simulink model "blance_leg2"  (R2021b)
settings: Solver=VariableStepAuto  StartTime=0.0  StopTime=10  RelTol=1e-3
values from neighbouring files (symbols this model uses):
  K = get_k_length(0.14)    [get_k.m]    (also in get_k_length.m = lqr(A,B,Q,R))
  N = NM + mp*diff(x + L*sin(theta),t,2)    [get_k_length.m]
undefined symbols (not defined in the file or in its folder): X, Y, Z
libraries: sm_lib x76, nesl_utility x25, slpidlib x2
(part 1 of 3)
settings Model: Creator=Hhop  LastModifiedBy=34511
settings SolverCC: AlgebraicLoopSolver=TrustRegion  MinimalZcImpactIntegration=on
settings DebuggingCC: ReadBeforeWriteMsg=DisableAll  WriteAfterWriteMsg=DisableAll  WriteAfterReadMsg=DisableAll  MultiTaskDSMMsg=none  UnconnectedInputMsg=none  UnconnectedOutputMsg=none  UnconnectedLineMsg=none
settings ModelReferenceCC: UpdateModelReferenceTargets=IfOutOfDate  EnableRefExpFcnMdlSchedulingChecks=off
settings SFSimCC: SFSimEcho=off

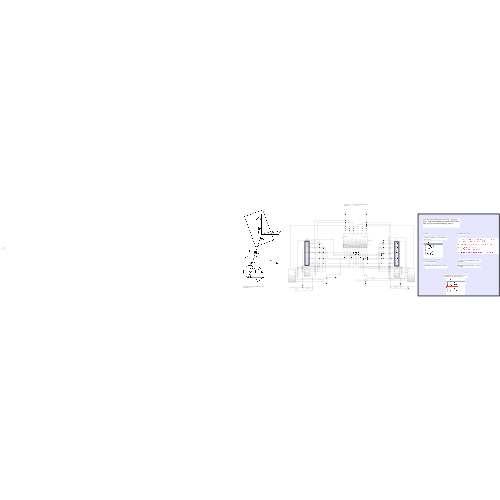
[thumbnail: Simulink's stored preview of the top-level diagram]
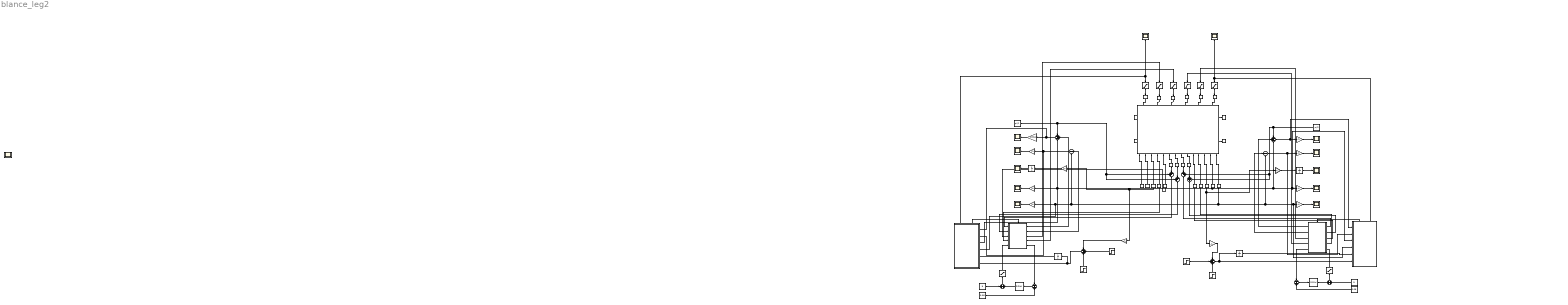
== system blance_leg2 ==
  note: 参考开源文档作者：韭菜的菜 链接：https://zhuanlan.zhihu.com/p/613007726 来源：知乎
  note: 图片来源 韭菜的菜 链接：https://zhuanlan.zhihu.com/p/613007726来源：知乎
  note: 运行步骤 :
  note: 所有开源文件必须置于同一文件夹(最好不要使用中文路径)
  note: 得到K参数后进入simulink 点击“运行”开始仿真
  note: addpath'(你所要想添加到的路径)'，具体用法可自行搜索
  note: 如果遇到如下图所示错误
  note: 可点击将其文件夹添加到MATLAB，或输入代码更换路径
  note: K = get_k_length(0.08)
  note: 在命令行窗口运行下图所示代码
  note: 如果想获取K矩阵关于腿长的函数的三次多项式系数在命令行窗口运行下图所示文件
  note: 该仿真是在b站轮腿机器人仿真开源上进行修改，链接：https://www.bilibili.com/read/cv26677904/?spm_id_from=333.999.0.0&jump_opus=1
  Constant : Constant  Value=0.08
  Constant1 : Constant  Value=0.08
  Constant10 : Constant  Value=pi/2
  Constant12 : Constant  Value=pi/2
  Gain{,1,29,41} (4 alike) : Gain  Gain=-0.0603
  Gain{22,24..26,33,36,38,40} (8 alike) : Gain  Gain=180/pi
  Integrator{1..4} (4 alike) : Integrator
  L_X : Scope
  L_d_phi : Scope
  L_d_theta : Scope
  L_phi : Scope
  L_theta : Scope
  PID Controller2 : slpidlib/PID Controller  Controller=PID  Form=Parallel  TimeDomain=Continuous-time  UseExternalTs=off  SampleTime=-1  IntegratorMethod=Forward Euler  FilterMethod=Forward Euler  ControllerParametersSource=internal  P=220  I=0  D=1000  UseFilter=on  N=100  TunerSelectOption=Transfer Function Based (PID Tuner App)  InitialConditionSource=internal  InitialConditionForIntegrator=0  InitialConditionForFilter=0  DifferentiatorICPrevScaledInput=0  ExternalReset=none  TrackingMode=off  Kt=1  LimitOutput=off  SatLimitsSource=internal  UpperSaturationLimit=inf  LowerSaturationLimit=-inf  LinearizeAsGain=on  AntiWindupMode=none  Kb=1  POutMin=[]  POutMax=[]  IOutMin=[]  IOutMax=[]  DOutMin=[]  DOutMax=[]  NOutMin=[]  NOutMax=[]  SumOutMin=[]  SumOutMax=[]  SaturationOutMin=[]  SaturationOutMax=[]  PParamMin=[]  PParamMax=[]  IParamMin=[]  IParamMax=[]  DParamMin=[]  DParamMax=[]  NParamMin=[]  NParamMax=[]  KbParamMin=[]  KbParamMax=[]  KtParamMin=[]  KtParamMax=[]  KbOutMin=[]  KbOutMax=[]  KtOutMin=[]  KtOutMax=[]  IntegratorOutMin=[]  IntegratorOutMax=[]  FilterOutMin=[]  FilterOutMax=[]  SumI1OutMin=[]  SumI1OutMax=[]  SumI2OutMin=[]  SumI2OutMax=[]  SumI3OutMin=[]  SumI3OutMax=[]  SumI4OutMin=[]  SumI4OutMax=[]  SumDOutMin=[]  SumDOutMax=[]  DifferentiatorOutMin=[]  DifferentiatorOutMax=[]  FilterDiffOutCoefMin=[]  FilterDiffOutCoefMax=[]  ReciprocalOutMin=[]  ReciprocalOutMax=[]  SumDenOutMin=[]  SumDenOutMax=[]  SumNumOutMin=[]  SumNumOutMax=[]  DivideOutMin=[]  DivideOutMax=[]  UdiffTsProdOutMin=[]  UdiffTsProdOutMax=[]  NTsProdOutMin=[]  NTsProdOutMax=[]  UintegralTsProdOutMin=[]  UintegralTsProdOutMax=[]  UngainTsProdOutMin=[]  UngainTsProdOutMax=[]  IntegratorContinuousStateAttributes=''  IntegratorStateMustResolveToSignalObject=off  IntegratorRTWStateStorageClass=Auto  FilterContinuousStateAttributes=''  FilterStateMustResolveToSignalObject=off  FilterRTWStateStorageClass=Auto  ParallelPVariant=InternalParameters  IdealPVariant=Disabled  IVariant=InternalParameters  DVariant=InternalParameters  IntegratorVariant=Continuous  SatVariant=Disabled  AWVariant=Passthrough  PCopyVariant=Disabled  TRVariant=Disabled  FdbkBlocksVariant=Forward  IdealPFdbkVariant=Disabled  SatFdbkVariant=Disabled  DerivativeFilterVariant=ContFilter  NVariant=InternalParameters  NCopyVariant=Disabled  FilterICVariant=InternalICsFilter  IntegratorICVariant=InternalICs  ExternalResetVariant=Disabled  TRSumVariant=Passthrough  SumFdbkVariant=Disabled  SumVariant=Sum_PID  TsampFilterVariant=InternalTs  TsampNgainVariant=Passthrough  TsampIntegralVariant=Passthrough  ExternalSaturationOutDataTypeStr=Inherit: Same as second input
  PID Controller3 : slpidlib/PID Controller  Controller=PID  Form=Parallel  TimeDomain=Continuous-time  UseExternalTs=off  SampleTime=-1  IntegratorMethod=Forward Euler  FilterMethod=Forward Euler  ControllerParametersSource=internal  P=220  I=0  D=1000  UseFilter=on  N=100  TunerSelectOption=Transfer Function Based (PID Tuner App)  InitialConditionSource=internal  InitialConditionForIntegrator=0  InitialConditionForFilter=0  DifferentiatorICPrevScaledInput=0  ExternalReset=none  TrackingMode=off  Kt=1  LimitOutput=off  SatLimitsSource=internal  UpperSaturationLimit=inf  LowerSaturationLimit=-inf  LinearizeAsGain=on  AntiWindupMode=none  Kb=1  POutMin=[]  POutMax=[]  IOutMin=[]  IOutMax=[]  DOutMin=[]  DOutMax=[]  NOutMin=[]  NOutMax=[]  SumOutMin=[]  SumOutMax=[]  SaturationOutMin=[]  SaturationOutMax=[]  PParamMin=[]  PParamMax=[]  IParamMin=[]  IParamMax=[]  DParamMin=[]  DParamMax=[]  NParamMin=[]  NParamMax=[]  KbParamMin=[]  KbParamMax=[]  KtParamMin=[]  KtParamMax=[]  KbOutMin=[]  KbOutMax=[]  KtOutMin=[]  KtOutMax=[]  IntegratorOutMin=[]  IntegratorOutMax=[]  FilterOutMin=[]  FilterOutMax=[]  SumI1OutMin=[]  SumI1OutMax=[]  SumI2OutMin=[]  SumI2OutMax=[]  SumI3OutMin=[]  SumI3OutMax=[]  SumI4OutMin=[]  SumI4OutMax=[]  SumDOutMin=[]  SumDOutMax=[]  DifferentiatorOutMin=[]  DifferentiatorOutMax=[]  FilterDiffOutCoefMin=[]  FilterDiffOutCoefMax=[]  ReciprocalOutMin=[]  ReciprocalOutMax=[]  SumDenOutMin=[]  SumDenOutMax=[]  SumNumOutMin=[]  SumNumOutMax=[]  DivideOutMin=[]  DivideOutMax=[]  UdiffTsProdOutMin=[]  UdiffTsProdOutMax=[]  NTsProdOutMin=[]  NTsProdOutMax=[]  UintegralTsProdOutMin=[]  UintegralTsProdOutMax=[]  UngainTsProdOutMin=[]  UngainTsProdOutMax=[]  IntegratorContinuousStateAttributes=''  IntegratorStateMustResolveToSignalObject=off  IntegratorRTWStateStorageClass=Auto  FilterContinuousStateAttributes=''  FilterStateMustResolveToSignalObject=off  FilterRTWStateStorageClass=Auto  ParallelPVariant=InternalParameters  IdealPVariant=Disabled  IVariant=InternalParameters  DVariant=InternalParameters  IntegratorVariant=Continuous  SatVariant=Disabled  AWVariant=Passthrough  PCopyVariant=Disabled  TRVariant=Disabled  FdbkBlocksVariant=Forward  IdealPFdbkVariant=Disabled  SatFdbkVariant=Disabled  DerivativeFilterVariant=ContFilter  NVariant=InternalParameters  NCopyVariant=Disabled  FilterICVariant=InternalICsFilter  IntegratorICVariant=InternalICs  ExternalResetVariant=Disabled  TRSumVariant=Passthrough  SumFdbkVariant=Disabled  SumVariant=Sum_PID  TsampFilterVariant=InternalTs  TsampNgainVariant=Passthrough  TsampIntegralVariant=Passthrough  ExternalSaturationOutDataTypeStr=Inherit: Same as second input
  PS-Simulink Converter{1,18..22,24,27..37} (18 alike) : nesl_utility/PS-Simulink Converter  PhysicalDomain=network_engine_domain  SubClassName=ps_output  LeftPortType=input  RightPortType=output  PseudoPeriodic=off  Frequencies=[]  Unit=inherit  AffineConversion=off
      settings: SourceProductBaseCode=PW,SS
  R_X : Scope
  R_d_phi : Scope
  R_d_theta : Scope
  R_phi : Scope
  R_theta : Scope
  Saturation{1..4} (4 alike) : Saturate  UpperLimit=100  LowerLimit=-100
  Saturation5 : Saturate  UpperLimit=300  LowerLimit=-300
  Saturation6 : Saturate  UpperLimit=300  LowerLimit=-300
  Saturation7 : Saturate  UpperLimit=9  LowerLimit=-9
  Saturation8 : Saturate  UpperLimit=9  LowerLimit=-9
  Scope1 : Scope
  Scope6 : Scope
  Simulink-PS Converter{1..6} (6 alike) : nesl_utility/Simulink-PS Converter  PhysicalDomain=network_engine_domain  SubClassName=ps_input  LeftPortType=input  RightPortType=output  PseudoPeriodic=off  Frequencies=[]  NoiseDistribution=none  NoiseParameters=[]  Unit=1  AffineConversion=off  FilteringAndDerivatives=provide  SimscapeFilterOrder=1  InputFilterTimeConstant=0.001  UdotUserProvided=0
      settings: SourceProductBaseCode=PW,SS
  Step1 : Step  Time=2  After=0.5  SampleTime=0
  Step5 : Step  Time=5  After=0.5  SampleTime=0
  Step6 : Step  Time=5  After=0.5  SampleTime=0
  Step7 : Step  Time=2  After=0.5  SampleTime=0
  Subsystem1 : Subsystem
      settings: PortSchema="{\"entries\":[{\"content\":{\"sides\":[{\"content\":{\"connectorIds\":[\"In1\",\"In2\",\"In3\",\"In4\",\"In5\",\"In6\"]},\"type\":\"ConnectorPlacement.EquallySpacedRectSide\",\"uuid\":\"055cb80c-cd03-4a8d-aef8-6b3df8c72d3f\"},{\"content\":{\"connectorIds\":[],\"side\":\"RIGHT\"},\"type\":\"ConnectorPlacement.EquallySpacedRectSide\",\"uuid\":\"5756fad1-d70f-4a11-a5af-d2f67bfb0d7e\"},{\"content\":{\"connectorIds\":[\"Out1\",\"Out2\"],\"side\":\"TOP\"},\"type\":\"ConnectorPlacement.EquallySpacedRectSide\",\"uuid\":\"9c70cf42-10f8-4525-9406-562484abf580\"}]},\"type\":\"ConnectorPlacement.EquallySpacedConnector\",\"uuid\":\"7084d402-0e44-4d2f-8cc2-1336d196e84d\"}],\"packageUris\":[\"http://schema.mathworks.com/mf0/Connector/R2020b\"],\"version\":\"1.0\"}"
  Subsystem4 : Subsystem
      settings: PortSchema="{\"entries\":[{\"content\":{\"sides\":[{\"content\":{\"connectorIds\":[\"In1\",\"In2\",\"In3\",\"In4\",\"In5\"]},\"type\":\"ConnectorPlacement.EquallySpacedRectSide\",\"uuid\":\"40de31e0-cc19-460f-99e9-affbb47f7204\"},{\"content\":{\"connectorIds\":[\"Out1\",\"Out2\",\"Out3\",\"Out4\",\"Out5\"],\"side\":\"RIGHT\"},\"type\":\"ConnectorPlacement.EquallySpacedRectSide\",\"uuid\":\"e61df4ab-633d-456a-aa2d-223df880274d\"},{\"content\":{\"connectorIds\":[\"In6\"],\"side\":\"TOP\"},\"type\":\"ConnectorPlacement.EquallySpacedRectSide\",\"uuid\":\"a7334146-3144-4ab1-9f08-8bf1583597b4\"}]},\"type\":\"ConnectorPlacement.EquallySpacedConnector\",\"uuid\":\"1490fe93-b025-4c86-96e6-b1bfc13c7f50\"}],\"packageUris\":[\"http://schema.mathworks.com/mf0/Connector/R2020b\"],\"version\":\"1.0\"}"
  Sum1 : Sum  Inputs=+-+
  Sum13 : Sum  Inputs=++|
  Sum14 : Sum  Inputs=|++
  Sum15 : Sum  Inputs=|++
  Sum16 : Sum  Inputs=|--
  Sum17 : Sum  Inputs=+--
  Sum18 : Sum  Inputs=+|+
  Sum2 : Sum  Inputs=+-+
  Sum20 : Sum  Inputs=++|
  Sum23 : Sum  Inputs=-|+
  Sum24 : Sum  Inputs=+--
  Sum25 : Sum  Inputs=+|+
  Sum27 : Sum  Inputs=|--
  Sum29 : Sum  Inputs=-|+
  blance_leg_model : Subsystem
      settings: PortSchema="{\"entries\":[{\"content\":{\"sides\":[{\"content\":{\"connectorIds\":[\"LConn1\",\"LConn2\",\"LConn3\",\"LConn4\",\"LConn5\",\"LConn6\"]},\"type\":\"ConnectorPlacement.EquallySpacedRectSide\",\"uuid\":\"df2d0b15-ec70-4430-8d90-67c6d88950b4\"},{\"content\":{\"connectorIds\":[\"RConn1\",\"RConn2\",\"RConn3\",\"RConn4\",\"RConn5\",\"RConn6\",\"RConn7\",\"RConn8\",\"RConn9\",\"RConn10\",\"RConn11\",\"RConn12\",\"RConn13\",\"RConn14\"],\"side\":\"RIGHT\"},\"type\":\"ConnectorPlacement.EquallySpacedRectSide\",\"uuid\":\"ec9b4787-d265-4ad9-b676-e253d2304993\"},{\"content\":{\"connectorIds\":[\"LConn7\",\"LConn8\"],\"side\":\"TOP\"},\"type\":\"ConnectorPlacement.EquallySpacedRectSide\",\"uuid\":\"40dd08fe-dc32-4cee-bbb8-c1ec6d04ee32\"},{\"content\":{\"connectorIds\":[\"RConn15\",\"RConn16\"],\"side\":\"BOTTOM\"},\"type\":\"ConnectorPlacement.EquallySpacedRectSide\",\"uuid\":\"0f9c1faf-3e52-4dca-bbb1-0993be9fa88c\"}]},\"type\":\"ConnectorPlacement.EquallySpacedConnector\",\"uuid\":\"d540d646-85aa-4f97-ae4d-1bccec971368\"}],\"packageUris\":[\"http://schema.mathworks.com/mf0/Connector/R2020b\"],\"version\":\"1.0\"}"
  calc : Subsystem
      settings: PortSchema="{\"entries\":[{\"content\":{\"sides\":[{\"content\":{\"connectorIds\":[\"In1\",\"In2\",\"In3\",\"In4\",\"In5\",\"In6\"]},\"type\":\"ConnectorPlacement.EquallySpacedRectSide\",\"uuid\":\"055cb80c-cd03-4a8d-aef8-6b3df8c72d3f\"},{\"content\":{\"connectorIds\":[],\"side\":\"RIGHT\"},\"type\":\"ConnectorPlacement.EquallySpacedRectSide\",\"uuid\":\"5756fad1-d70f-4a11-a5af-d2f67bfb0d7e\"},{\"content\":{\"connectorIds\":[\"Out1\",\"Out2\"],\"side\":\"TOP\"},\"type\":\"ConnectorPlacement.EquallySpacedRectSide\",\"uuid\":\"9c70cf42-10f8-4525-9406-562484abf580\"}]},\"type\":\"ConnectorPlacement.EquallySpacedConnector\",\"uuid\":\"7084d402-0e44-4d2f-8cc2-1336d196e84d\"}],\"packageUris\":[\"http://schema.mathworks.com/mf0/Connector/R2020b\"],\"version\":\"1.0\"}"
  control : Subsystem
      settings: PortSchema="{\"entries\":[{\"content\":{\"sides\":[{\"content\":{\"connectorIds\":[\"In1\",\"In2\",\"In3\",\"In4\",\"In5\"]},\"type\":\"ConnectorPlacement.EquallySpacedRectSide\",\"uuid\":\"40de31e0-cc19-460f-99e9-affbb47f7204\"},{\"content\":{\"connectorIds\":[\"Out1\",\"Out2\",\"Out3\",\"Out4\",\"Out5\"],\"side\":\"RIGHT\"},\"type\":\"ConnectorPlacement.EquallySpacedRectSide\",\"uuid\":\"e61df4ab-633d-456a-aa2d-223df880274d\"},{\"content\":{\"connectorIds\":[\"In6\"],\"side\":\"TOP\"},\"type\":\"ConnectorPlacement.EquallySpacedRectSide\",\"uuid\":\"a7334146-3144-4ab1-9f08-8bf1583597b4\"}]},\"type\":\"ConnectorPlacement.EquallySpacedConnector\",\"uuid\":\"1490fe93-b025-4c86-96e6-b1bfc13c7f50\"}],\"packageUris\":[\"http://schema.mathworks.com/mf0/Connector/R2020b\"],\"version\":\"1.0\"}"
  mean_x2 : Scope
  除去轮子后机体重量 : Constant  Value=9
  除去轮子后机体重量， : Constant  Value=9
  wires:
  Integrator4/1 -> R_X/1  "x"
  Integrator2/1 -> L_X/1  "x"
  除去轮子后机体重量，/1 -> Sum25/1
  Sum27/1 -> Subsystem1/2(d_theta), Gain25/1
  Gain40/1 -> L_d_phi/1
  Gain24/1 -> R_theta/1
  Gain38/1 -> L_d_theta/1
  Constant12/1 -> Sum15/2, Sum14/2, Sum17/1
  Sum29/1 -> PID Controller3/1
  Gain33/1 -> R_phi/1
  Gain36/1 -> L_theta/1
  Gain41/1 -> Integrator2/1  "x'"
  Sum16/1 -> calc/2(d_theta), Gain38/1
  Gain26/1 -> R_d_phi/1
  Constant/1 -> Sum29/2
  Gain22/1 -> L_phi/1
  Sum24/1 -> calc/1(theta), Gain36/1
  Constant10/1 -> Sum20/1, Sum13/1, Sum24/1
  Gain29/1 -> Integrator4/1  "x'"
  Sum23/1 -> PID Controller2/1
  PID Controller2/1 -> Sum25/2
  Sum17/1 -> Subsystem1/1(theta), Gain24/1
  Gain25/1 -> R_d_theta/1
  除去轮子后机体重量/1 -> Sum18/2
  PID Controller3/1 -> Sum18/1
  Saturation1/1 -> Simulink-PS Converter1/1
  Saturation2/1 -> Simulink-PS Converter3/1
  Saturation3/1 -> Simulink-PS Converter2/1
  Saturation4/1 -> Simulink-PS Converter5/1
  PS-Simulink Converter32/1 -> Sum13/2
  PS-Simulink Converter35/1 -> Sum15/1
  PS-Simulink Converter33/1 -> Sum14/1
  PS-Simulink Converter34/1 -> Sum20/2
  Sum13/1 -> control/1(phi1)
  Sum20/1 -> control/2(phi4)
  Sum14/1 -> Subsystem4/1(phi1)
  Sum15/1 -> Subsystem4/2(phi4)
  PS-Simulink Converter31/1 -> control/3(d_phi1)
  PS-Simulink Converter29/1 -> control/4(d_phi4)
  PS-Simulink Converter20/1 -> Subsystem4/3(d_phi1)
  PS-Simulink Converter21/1 -> Subsystem4/4(d_phi4)
  PS-Simulink Converter28/1 -> Gain41/1, Gain1/1
  PS-Simulink Converter22/1 -> Gain29/1, Gain/1
  PS-Simulink Converter1/1 -> calc/3(phi), Gain22/1, Sum24/3, Subsystem1/3(phi), Gain33/1, Sum17/3
  PS-Simulink Converter24/1 -> calc/4(d_phi), Gain40/1, Sum16/2, Subsystem1/4(d_phi), Gain26/1, Sum27/2
  control/5(L0) -> Sum23/1
  control/1(phi0) -> Sum24/2
  control/2(d_phi0) -> Sum16/1
  Subsystem4/1(phi0) -> Sum17/2
  Subsystem4/2(d_phi0) -> Sum27/1
  Subsystem4/5(L0) -> Sum29/1
  calc/1(Tp) -> control/6(Tp)
  Sum18/1 -> Saturation5/1
  Sum25/1 -> Saturation6/1
  Saturation6/1 -> control/5(F0)
  Constant1/1 -> Sum23/2
  control/3(T1) -> Saturation1/1
  Subsystem4/3(T1) -> Saturation4/1
  control/4(T2) -> Saturation2/1
  Subsystem4/4(T2) -> Saturation3/1
  calc/2(T) -> Saturation7/1, Scope1/1
  Subsystem1/2(T) -> Saturation8/1, Scope6/1
  Saturation7/1 -> Simulink-PS Converter6/1
  Saturation8/1 -> Simulink-PS Converter4/1
  Integrator1/1 -> Subsystem1/5(x)
  Integrator3/1 -> calc/5(x)
  Gain1/1 -> Sum1/1
  Sum1/1 -> calc/6(d_x), Integrator3/1
  Gain/1 -> Sum2/1
  Sum2/1 -> Integrator1/1, Subsystem1/6(d_x)
  Step1/1 -> Sum1/2
  Step5/1 -> Sum1/3
  Step7/1 -> Sum2/2
  Step6/1 -> Sum2/3
  Subsystem1/1(Tp) -> Subsystem4/6(Tp)
  Saturation5/1 -> Subsystem4/5(F0)
  connections:
  blance_leg_model/LConn2 -- Simulink-PS Converter1/RConn1
  blance_leg_model/LConn3 -- Simulink-PS Converter3/RConn1
  blance_leg_model/LConn4 -- Simulink-PS Converter2/RConn1
  blance_leg_model/LConn5 -- Simulink-PS Converter5/RConn1
  blance_leg_model/RConn10 -- PS-Simulink Converter20/LConn1
  blance_leg_model/RConn11 -- PS-Simulink Converter21/LConn1
  blance_leg_model/RConn2 -- PS-Simulink Converter19/LConn1
  blance_leg_model/RConn12 -- PS-Simulink Converter22/LConn1
  blance_leg_model/RConn3 -- PS-Simulink Converter28/LConn1
  blance_leg_model/RConn14 -- PS-Simulink Converter24/LConn1
  blance_leg_model/RConn5 -- PS-Simulink Converter31/LConn1
  blance_leg_model/RConn1 -- PS-Simulink Converter18/LConn1
  blance_leg_model/RConn4 -- PS-Simulink Converter29/LConn1
  blance_leg_model/RConn13 -- PS-Simulink Converter1/LConn1
  blance_leg_model/RConn6 -- PS-Simulink Converter32/LConn1
  blance_leg_model/RConn7 -- PS-Simulink Converter34/LConn1
  blance_leg_model/RConn8 -- PS-Simulink Converter33/LConn1
  blance_leg_model/RConn9 -- PS-Simulink Converter35/LConn1
  blance_leg_model/LConn7 -- PS-Simulink Converter27/LConn1
  blance_leg_model/LConn8 -- PS-Simulink Converter30/LConn1
  blance_leg_model/RConn15 -- PS-Simulink Converter36/LConn1
  blance_leg_model/RConn16 -- PS-Simulink Converter37/LConn1
  blance_leg_model/LConn1 -- Simulink-PS Converter6/RConn1
  blance_leg_model/LConn6 -- Simulink-PS Converter4/RConn1

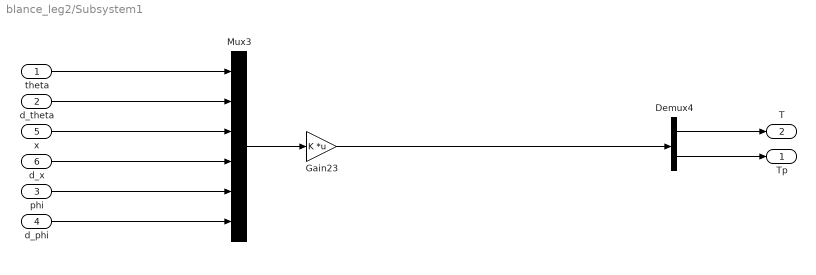
== system blance_leg2/Subsystem1 ==
  theta : Inport
  d_theta : Inport  Port=2
  phi : Inport  Port=3
  d_phi : Inport  Port=4
  x : Inport  Port=5
  d_x : Inport  Port=6
  Demux4 : Demux  Outputs=2
  Gain23 : Gain  Gain=K  Multiplication=Matrix(K*u) (u vector)
  Mux3 : Mux  Inputs=6
  Tp : Outport
  T : Outport  Port=2
  wires:
  theta/1 -> Mux3/1
  d_theta/1 -> Mux3/2
  d_x/1 -> Mux3/4
  d_phi/1 -> Mux3/6
  phi/1 -> Mux3/5
  Demux4/2 -> Tp/1
  x/1 -> Mux3/3
  Mux3/1 -> Gain23/1
  Gain23/1 -> Demux4/1
  Demux4/1 -> T/1

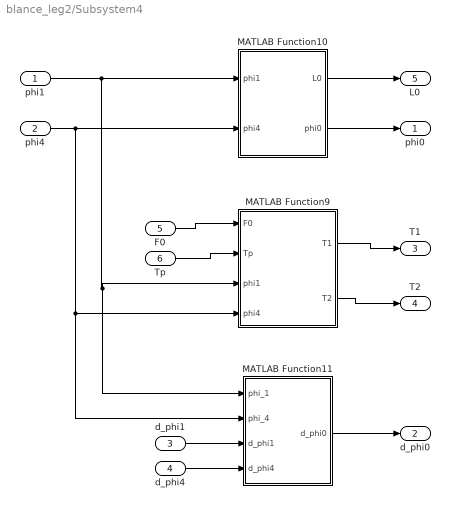
== system blance_leg2/Subsystem4 ==
  phi1 : Inport
  phi4 : Inport  Port=2
  d_phi1 : Inport  Port=3
  d_phi4 : Inport  Port=4
  F0 : Inport  Port=5
  Tp : Inport  Port=6
  MATLAB Function10 : MATLAB Function  TreatAsAtomicUnit=on
  MATLAB Function11 : MATLAB Function  TreatAsAtomicUnit=on
  MATLAB Function9 : MATLAB Function  TreatAsAtomicUnit=on
  phi0 : Outport
  d_phi0 : Outport  Port=2
  T1 : Outport  Port=3
  T2 : Outport  Port=4
  L0 : Outport  Port=5
  wires:
  phi1/1 -> MATLAB Function11/1(phi_1), MATLAB Function9/3(phi1), MATLAB Function10/1(phi1)
  MATLAB Function10/2(phi0) -> phi0/1
  MATLAB Function11/1(d_phi0) -> d_phi0/1
  Tp/1 -> MATLAB Function9/2(Tp)
  d_phi4/1 -> MATLAB Function11/4(d_phi4)
  d_phi1/1 -> MATLAB Function11/3(d_phi1)
  MATLAB Function9/1(T1) -> T1/1
  phi4/1 -> MATLAB Function11/2(phi_4), MATLAB Function9/4(phi4), MATLAB Function10/2(phi4)
  F0/1 -> MATLAB Function9/1(F0)
  MATLAB Function9/2(T2) -> T2/1
  MATLAB Function10/1(L0) -> L0/1
